simulink model "EVSR24"  (R2022b)
settings: Solver=VariableStepAuto  StartTime=0.0  StopTime=10.0  RelTol=1e-3
undefined symbols (not defined in the file): BattPwrChrgLim, BattPwrDischrgLim, BrkCmd, MotTrqCmdRegen
settings Model: Creator=serga  LastModifiedBy=serga

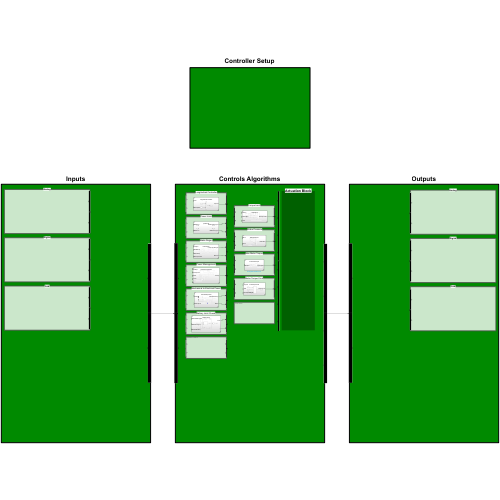
[thumbnail: Simulink's stored preview of the top-level diagram]
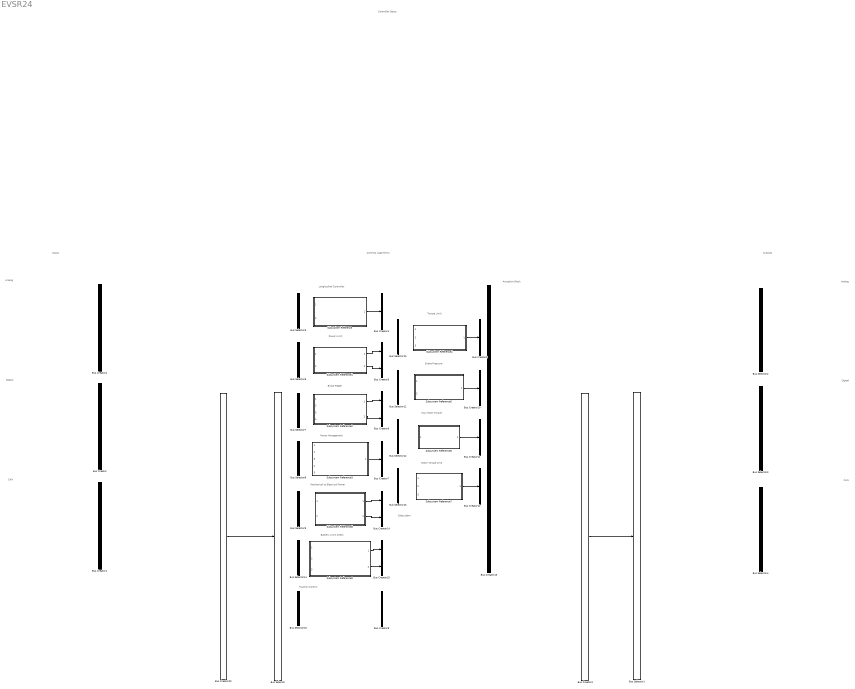
== system EVSR24 ==
  note: Longitudinal Controller
  note: Controls Algorithms
  note: Subsystem
  note: Power Limit
  note: Brake Regen
  note: Power Management
  note: Torque Limit
  note: Brake Pressure
  note: Outputs
  note: Inputs
  note: Controller Setup
  note: Analog
  note: Digital
  note: CAN
  note: Analog
  note: Digital
  note: CAN
  note: Actuation Block
  note: Max Motor Torque
  note: Motor Torque Cmd
  note: Mechanical to Electrical Power
  note: Traction Control
  note: Battery Limit Check
  Bus Creator{,1..2,8,14..15,20} (7 alike) : BusCreator  Inputs=2
  Bus Creator10 : BusCreator  Inputs=BrkPrsReq
  Bus Creator11 : BusCreator  Inputs=MotTrqMax
  Bus Creator12 : BusCreator  Inputs=MotTrqCmd
  Bus Creator13 : BusCreator  Inputs=8
  Bus Creator3 : BusCreator  Inputs=4
  Bus Creator4 : BusCreator  Inputs=TrqCmd
  Bus Creator5 : BusCreator  Inputs=BattPwrDischrgLim,BattPwrChrgLim
  Bus Creator6 : BusCreator  Inputs=MotTrqCmdRegen,BrkCmd
  Bus Creator7 : BusCreator  Inputs=MotTrqCmdFnl
  Bus Creator9 : BusCreator  Inputs=MotTrqCmdFnl
  Bus Selector{,1..15} (16 alike) : BusSelector  OutputSignals=signal1,signal2
  Subsystem Reference : Subsystem  ReferencedSubsystem=longitudinalcontroller
  Subsystem Reference1 : Subsystem  ReferencedSubsystem=powerlimit
  Subsystem Reference2 : Subsystem  ReferencedSubsystem=brakeregen
  Subsystem Reference3 : Subsystem  ReferencedSubsystem=powermanagement
  Subsystem Reference4 : Subsystem  ReferencedSubsystem=torquelimit
  Subsystem Reference5 : Subsystem  ReferencedSubsystem=brakepressure
  Subsystem Reference6 : Subsystem  ReferencedSubsystem=motormaxtorque
  Subsystem Reference7 : Subsystem  ReferencedSubsystem=motortorquecmd
  Subsystem Reference8 : Subsystem  ReferencedSubsystem=mechtoelecpower
  Subsystem Reference9 : Subsystem  ReferencedSubsystem=battlimcheck
  wires:
  Bus Creator3/1 -> Bus Selector1/1
  Subsystem Reference4/1 -> Bus Creator9/1
  Subsystem Reference1/1 -> Bus Creator5/1
  Subsystem Reference2/1 -> Bus Creator6/1
  Subsystem Reference2/2 -> Bus Creator6/2
  Subsystem Reference3/1 -> Bus Creator7/1
  Subsystem Reference/1 -> Bus Creator4/1
  Subsystem Reference5/1 -> Bus Creator10/1
  Subsystem Reference6/1 -> Bus Creator11/1
  Subsystem Reference7/1 -> Bus Creator12/1
  Bus Creator20/1 -> Bus Selector/1
  Subsystem Reference1/2 -> Bus Creator5/2
  Subsystem Reference8/1 -> Bus Creator14/1
  Subsystem Reference8/2 -> Bus Creator14/2
  Subsystem Reference9/1 -> Bus Creator15/1
  Subsystem Reference9/2 -> Bus Creator15/2
